simulink model "pd_path_sg"  (R2013b)
settings: Solver=ode45  StartTime=0.0  StopTime=10  RelTol=1e-3
undefined symbols (not defined in the file or in its folder): A, A2, B, C, D, EVAL, i, output_samp_bcoef, PCIN, reg_pk_lim, reg_plim, reg_scale, reg_sr_lim, reg_staclr, reg_txgain, THIS_DATE, W, X, Z
undefined symbols (not defined in the file): lut_address, lut_address_s5, reg_dltap
libraries: xbsIndex_r4 x3819, lut_ram_vhdl x32
(part 10 of 31)

== system pd_path_sg/gmp_model_B/cmp_mul5 ==
  x : Inport
  coef : Inport  Port=2
  pcin_i : Inport  Port=3
  pcin_q : Inport  Port=4
  Convert{10,12,15..16} (4 alike) : xbsIndex_r4/Convert  gui_display_data_type=Fixed-point  arith_type="Signed  (2's comp)"  n_bits=30  bin_pt=0  float_type=Single  exp_bits=8  fraction_bits=24  quantization=Truncate  overflow=Wrap  en=off  latency=0  pipeline=off  dbl_ovrd=off  block_type=convert
  Convert{11,13..14,17} (4 alike) : xbsIndex_r4/Convert  gui_display_data_type=Fixed-point  arith_type="Signed  (2's comp)"  n_bits=18  bin_pt=0  float_type=Single  exp_bits=8  fraction_bits=24  quantization=Truncate  overflow=Wrap  en=off  latency=0  pipeline=off  dbl_ovrd=off  block_type=convert
  "DSP48E2 " : xbsIndex_r4/DSP48E2   use_a=Direct from A Port  use_b=Direct from B Port  addsub_mode=ONE48  xl_useadderonly=off  xl_dynamicmult=off  preaddinsel=A  amultsel=A  bmultsel=B  enable_d=off  reset_preg=off  auto_reset_pr=RESET  pattern_from_creg=1  pattern='000000000000'  mask_from_creg=1  pattern_mask='000000000000'  rnd='000000000000'  widexor=off  xormode=1  use_op=on  use_creg=off  rst_all=off  en_all=off  use_pcin=on  use_carrycascin=off  use_multsignin=off  use_carryout=off  use_patterndetect=off  use_patternbdetect=off  use_overflow=off  use_underflow=off  use_acout=off  use_bcout=off  use_pcout=on  use_multsignout=off  use_carrycascout=off  pipeline_a=2  pipeline_b=2  pipeline_acout=1  pipeline_bcout=1  pipeline_c=on  pipeline_p=on  pipeline_mult=on  pipeline_opmode=on  pipeline_alumode=on  pipeline_carryin=on  pipeline_carryinsel=on  dreg=off  adreg=off  register_inmode=on  rst_a=off  rst_b=off  rst_c=off  rst_mult=off  rst_p=off  rst_carry_in=off  rst_alumode=off  rst_ctrl=off  reset_port_d=off  reset_port_inmode=off  en_a1=off  en_a2=off  en_b1=off  en_b2=off  en_c=off  en_mult=off  en_p=off  en_carry_in=off  en_alumode=off  en_multcarryin=off  en_ctrl=off  enable_port_regd=off  enable_port_regad=off  enable_port_reginmode=off  alumode_inverted=off  alumode_inverted_value='0000'  is_carryin_inverted=off  inmode_inverted=off  inmode_inverted_value='00000'  opmode_inverted=off  opmode_inverted_value='000000000'  is_rstallcarryin_inverted=off  is_rstalumode_inverted=off  is_rsta_inverted=off  is_rstb_inverted=off  is_rstc_inverted=off  is_rstd_inverted=off  is_rstctrl_inverted=off  is_rstinmode_inverted=off  is_rstm_inverted=off  is_rstp_inverted=off  use_synth_model=off  is_clk_inverted=false  block_type=dsp48e2
  DSP48E2 1 : xbsIndex_r4/DSP48E2   use_a=Direct from A Port  use_b=Direct from B Port  addsub_mode=ONE48  xl_useadderonly=off  xl_dynamicmult=off  preaddinsel=A  amultsel=A  bmultsel=B  enable_d=off  reset_preg=off  auto_reset_pr=RESET  pattern_from_creg=1  pattern='000000000000'  mask_from_creg=1  pattern_mask='000000000000'  rnd='000000000000'  widexor=off  xormode=1  use_op=on  use_creg=off  rst_all=off  en_all=off  use_pcin=on  use_carrycascin=off  use_multsignin=off  use_carryout=off  use_patterndetect=off  use_patternbdetect=off  use_overflow=off  use_underflow=off  use_acout=off  use_bcout=off  use_pcout=on  use_multsignout=off  use_carrycascout=off  pipeline_a=1  pipeline_b=1  pipeline_acout=1  pipeline_bcout=1  pipeline_c=on  pipeline_p=on  pipeline_mult=on  pipeline_opmode=on  pipeline_alumode=on  pipeline_carryin=on  pipeline_carryinsel=on  dreg=off  adreg=off  register_inmode=on  rst_a=off  rst_b=off  rst_c=off  rst_mult=off  rst_p=off  rst_carry_in=off  rst_alumode=off  rst_ctrl=off  reset_port_d=off  reset_port_inmode=off  en_a1=off  en_a2=off  en_b1=off  en_b2=off  en_c=off  en_mult=off  en_p=off  en_carry_in=off  en_alumode=off  en_multcarryin=off  en_ctrl=off  enable_port_regd=off  enable_port_regad=off  enable_port_reginmode=off  alumode_inverted=off  alumode_inverted_value='0000'  is_carryin_inverted=off  inmode_inverted=off  inmode_inverted_value='00000'  opmode_inverted=off  opmode_inverted_value='000000000'  is_rstallcarryin_inverted=off  is_rstalumode_inverted=off  is_rsta_inverted=off  is_rstb_inverted=off  is_rstc_inverted=off  is_rstd_inverted=off  is_rstctrl_inverted=off  is_rstinmode_inverted=off  is_rstm_inverted=off  is_rstp_inverted=off  use_synth_model=off  is_clk_inverted=false  block_type=dsp48e2
  DSP48E2 2 : xbsIndex_r4/DSP48E2   use_a=Direct from A Port  use_b=Direct from B Port  addsub_mode=ONE48  xl_useadderonly=off  xl_dynamicmult=off  preaddinsel=A  amultsel=A  bmultsel=B  enable_d=off  reset_preg=off  auto_reset_pr=RESET  pattern_from_creg=1  pattern='000000000000'  mask_from_creg=1  pattern_mask='000000000000'  rnd='000000000000'  widexor=off  xormode=1  use_op=on  use_creg=off  rst_all=off  en_all=off  use_pcin=on  use_carrycascin=off  use_multsignin=off  use_carryout=off  use_patterndetect=off  use_patternbdetect=off  use_overflow=off  use_underflow=off  use_acout=off  use_bcout=off  use_pcout=on  use_multsignout=off  use_carrycascout=off  pipeline_a=2  pipeline_b=2  pipeline_acout=1  pipeline_bcout=1  pipeline_c=on  pipeline_p=on  pipeline_mult=on  pipeline_opmode=on  pipeline_alumode=on  pipeline_carryin=on  pipeline_carryinsel=on  dreg=off  adreg=off  register_inmode=on  rst_a=off  rst_b=off  rst_c=off  rst_mult=off  rst_p=off  rst_carry_in=off  rst_alumode=off  rst_ctrl=off  reset_port_d=off  reset_port_inmode=off  en_a1=off  en_a2=off  en_b1=off  en_b2=off  en_c=off  en_mult=off  en_p=off  en_carry_in=off  en_alumode=off  en_multcarryin=off  en_ctrl=off  enable_port_regd=off  enable_port_regad=off  enable_port_reginmode=off  alumode_inverted=off  alumode_inverted_value='0000'  is_carryin_inverted=off  inmode_inverted=off  inmode_inverted_value='00000'  opmode_inverted=off  opmode_inverted_value='000000000'  is_rstallcarryin_inverted=off  is_rstalumode_inverted=off  is_rsta_inverted=off  is_rstb_inverted=off  is_rstc_inverted=off  is_rstd_inverted=off  is_rstctrl_inverted=off  is_rstinmode_inverted=off  is_rstm_inverted=off  is_rstp_inverted=off  use_synth_model=off  is_clk_inverted=false  block_type=dsp48e2
  DSP48E2 3 : xbsIndex_r4/DSP48E2   use_a=Direct from A Port  use_b=Direct from B Port  addsub_mode=ONE48  xl_useadderonly=off  xl_dynamicmult=off  preaddinsel=A  amultsel=A  bmultsel=B  enable_d=off  reset_preg=off  auto_reset_pr=RESET  pattern_from_creg=1  pattern='000000000000'  mask_from_creg=1  pattern_mask='000000000000'  rnd='000000000000'  widexor=off  xormode=1  use_op=on  use_creg=off  rst_all=off  en_all=off  use_pcin=on  use_carrycascin=off  use_multsignin=off  use_carryout=off  use_patterndetect=off  use_patternbdetect=off  use_overflow=off  use_underflow=off  use_acout=off  use_bcout=off  use_pcout=on  use_multsignout=off  use_carrycascout=off  pipeline_a=1  pipeline_b=1  pipeline_acout=1  pipeline_bcout=1  pipeline_c=on  pipeline_p=on  pipeline_mult=on  pipeline_opmode=on  pipeline_alumode=on  pipeline_carryin=on  pipeline_carryinsel=on  dreg=off  adreg=off  register_inmode=on  rst_a=off  rst_b=off  rst_c=off  rst_mult=off  rst_p=off  rst_carry_in=off  rst_alumode=off  rst_ctrl=off  reset_port_d=off  reset_port_inmode=off  en_a1=off  en_a2=off  en_b1=off  en_b2=off  en_c=off  en_mult=off  en_p=off  en_carry_in=off  en_alumode=off  en_multcarryin=off  en_ctrl=off  enable_port_regd=off  enable_port_regad=off  enable_port_reginmode=off  alumode_inverted=off  alumode_inverted_value='0000'  is_carryin_inverted=off  inmode_inverted=off  inmode_inverted_value='00000'  opmode_inverted=off  opmode_inverted_value='000000000'  is_rstallcarryin_inverted=off  is_rstalumode_inverted=off  is_rsta_inverted=off  is_rstb_inverted=off  is_rstc_inverted=off  is_rstd_inverted=off  is_rstctrl_inverted=off  is_rstinmode_inverted=off  is_rstm_inverted=off  is_rstp_inverted=off  use_synth_model=off  is_clk_inverted=false  block_type=dsp48e2
  Delay{1..4} (4 alike) : xbsIndex_r4/Delay  rst=off  infoeditControl=Selection of Reset will increase slice count due to use of real FFs and instead of SRLs  en=off  latency=10  reg_retiming=off  dbl_ovrd=off  block_type=delay
      settings: infoedit=Hardware notes: A delay line is a chain, each link of which is an SRL16 or SRL32 followed by a flip-flop.
  Demux : Demux  Outputs=2
  Demux1 : Demux  Outputs=2
  Null_p : xbsIndex_r4/Constant  const=0  gui_display_data_type=Fixed-point  arith_type=Unsigned  n_bits=16  bin_pt=0  preci_type=Single  exp_width=8  frac_width=24  explicit_period=off  period=1  equ=P=C  opselect=C  inp2=PCIN>>17  opr=+  inp1=P  carry=CIN  dbl_ovrd=off  block_type=constant
  Null_p1 : xbsIndex_r4/Constant  const=0  gui_display_data_type=Fixed-point  arith_type=Unsigned  n_bits=16  bin_pt=0  preci_type=Single  exp_width=8  frac_width=24  explicit_period=off  period=1  equ=P=C  opselect=C  inp2=PCIN>>17  opr=+  inp1=P  carry=CIN  dbl_ovrd=off  block_type=constant
  Opmode : xbsIndex_r4/Opmode  device=DSP48E2  equ=P=PCIN+(A*B)  operation=PCIN + A*B  inmode_0_3=D+A2  inmode_1_3=A*B  preaddinsel=A  amultsel=A  bmultsel=B  inmode_0=A2  inmode_4=B2  logicinstr=X + W + Z  z_mux=0  xy_mux=A*B  w_mux=RND  carry=0  dbl_ovrd=off  operand=+  x_mux=P  block_type=opmode
  Opmode1 : xbsIndex_r4/Opmode  device=DSP48E2  equ=P=PCIN-(A*B)  operation=Custom  inmode_0_3=D+A2  inmode_1_3=A*B  preaddinsel=A  amultsel=A  bmultsel=B  inmode_0=A2  inmode_4=B2  logicinstr=Z - (X + W)  z_mux=PCIN  xy_mux=A*B  w_mux=0  carry=0  dbl_ovrd=off  operand=+  x_mux=P  block_type=opmode
  Opmode2 : xbsIndex_r4/Opmode  device=DSP48E2  equ=P=PCIN+(A*B)  operation=Custom  inmode_0_3=D+A2  inmode_1_3=A*B  preaddinsel=A  amultsel=A  bmultsel=B  inmode_0=A2  inmode_4=B2  logicinstr=X + W + Z  z_mux=PCIN  xy_mux=A*B  w_mux=0  carry=0  dbl_ovrd=off  operand=+  x_mux=P  block_type=opmode
  Opmode3 : xbsIndex_r4/Opmode  device=DSP48E2  equ=P=PCIN+(A*B)  operation=PCIN + A*B  inmode_0_3=D+A2  inmode_1_3=A*B  preaddinsel=A  amultsel=A  bmultsel=B  inmode_0=A2  inmode_4=B2  logicinstr=X + W + Z  z_mux=PCIN  xy_mux=A*B  w_mux=0  carry=0  dbl_ovrd=off  operand=+  x_mux=P  block_type=opmode
  Terminator{,1..3} (4 alike) : Terminator
  no_route : Outport
  no_route1 : Outport  Port=2
  pcout_i : Outport  Port=3
  pcout_q : Outport  Port=4
  wires:
  Null_p1/1 -> no_route1/1
  Null_p/1 -> no_route/1
  Opmode1/1 -> "DSP48E2 "/4
  Opmode2/1 -> DSP48E2 2/4
  Opmode3/1 -> DSP48E2 3/4
  Opmode/1 -> DSP48E2 1/4
  Delay4/1 -> Convert17/1, Convert13/1
  Delay3/1 -> Convert11/1, Convert14/1
  Delay1/1 -> Convert15/1, Convert12/1
  Delay2/1 -> Convert16/1, Convert10/1
  coef/1 -> Demux1/1
  x/1 -> Demux/1
  Convert12/1 -> "DSP48E2 "/1
  Convert13/1 -> "DSP48E2 "/2
  Convert10/1 -> DSP48E2 1/1
  Convert14/1 -> DSP48E2 1/2
  DSP48E2 1/2 -> "DSP48E2 "/3
  Convert16/1 -> DSP48E2 2/1
  Convert17/1 -> DSP48E2 2/2
  Convert15/1 -> DSP48E2 3/1
  Convert11/1 -> DSP48E2 3/2
  DSP48E2 3/2 -> DSP48E2 2/3
  Demux1/1 -> Delay2/1
  Demux1/2 -> Delay1/1
  Demux/1 -> Delay3/1
  Demux/2 -> Delay4/1
  DSP48E2 1/1 -> Terminator/1
  DSP48E2 3/1 -> Terminator1/1
  DSP48E2 2/2 -> pcout_q/1
  "DSP48E2 "/2 -> pcout_i/1
  "DSP48E2 "/1 -> Terminator2/1
  DSP48E2 2/1 -> Terminator3/1
  pcin_i/1 -> DSP48E2 1/3
  pcin_q/1 -> DSP48E2 3/3

== system pd_path_sg/gmp_model_B/cmp_mul6 ==
  x : Inport
  coef : Inport  Port=2
  pcin_i : Inport  Port=3
  pcin_q : Inport  Port=4
  Convert{10,12,15..16} (4 alike) : xbsIndex_r4/Convert  gui_display_data_type=Fixed-point  arith_type="Signed  (2's comp)"  n_bits=30  bin_pt=0  float_type=Single  exp_bits=8  fraction_bits=24  quantization=Truncate  overflow=Wrap  en=off  latency=0  pipeline=off  dbl_ovrd=off  block_type=convert
  Convert{11,13..14,17} (4 alike) : xbsIndex_r4/Convert  gui_display_data_type=Fixed-point  arith_type="Signed  (2's comp)"  n_bits=18  bin_pt=0  float_type=Single  exp_bits=8  fraction_bits=24  quantization=Truncate  overflow=Wrap  en=off  latency=0  pipeline=off  dbl_ovrd=off  block_type=convert
  "DSP48E2 " : xbsIndex_r4/DSP48E2   use_a=Direct from A Port  use_b=Direct from B Port  addsub_mode=ONE48  xl_useadderonly=off  xl_dynamicmult=off  preaddinsel=A  amultsel=A  bmultsel=B  enable_d=off  reset_preg=off  auto_reset_pr=RESET  pattern_from_creg=1  pattern='000000000000'  mask_from_creg=1  pattern_mask='000000000000'  rnd='000000000000'  widexor=off  xormode=1  use_op=on  use_creg=off  rst_all=off  en_all=off  use_pcin=on  use_carrycascin=off  use_multsignin=off  use_carryout=off  use_patterndetect=off  use_patternbdetect=off  use_overflow=off  use_underflow=off  use_acout=off  use_bcout=off  use_pcout=on  use_multsignout=off  use_carrycascout=off  pipeline_a=2  pipeline_b=2  pipeline_acout=1  pipeline_bcout=1  pipeline_c=on  pipeline_p=on  pipeline_mult=on  pipeline_opmode=on  pipeline_alumode=on  pipeline_carryin=on  pipeline_carryinsel=on  dreg=off  adreg=off  register_inmode=on  rst_a=off  rst_b=off  rst_c=off  rst_mult=off  rst_p=off  rst_carry_in=off  rst_alumode=off  rst_ctrl=off  reset_port_d=off  reset_port_inmode=off  en_a1=off  en_a2=off  en_b1=off  en_b2=off  en_c=off  en_mult=off  en_p=off  en_carry_in=off  en_alumode=off  en_multcarryin=off  en_ctrl=off  enable_port_regd=off  enable_port_regad=off  enable_port_reginmode=off  alumode_inverted=off  alumode_inverted_value='0000'  is_carryin_inverted=off  inmode_inverted=off  inmode_inverted_value='00000'  opmode_inverted=off  opmode_inverted_value='000000000'  is_rstallcarryin_inverted=off  is_rstalumode_inverted=off  is_rsta_inverted=off  is_rstb_inverted=off  is_rstc_inverted=off  is_rstd_inverted=off  is_rstctrl_inverted=off  is_rstinmode_inverted=off  is_rstm_inverted=off  is_rstp_inverted=off  use_synth_model=off  is_clk_inverted=false  block_type=dsp48e2
  DSP48E2 1 : xbsIndex_r4/DSP48E2   use_a=Direct from A Port  use_b=Direct from B Port  addsub_mode=ONE48  xl_useadderonly=off  xl_dynamicmult=off  preaddinsel=A  amultsel=A  bmultsel=B  enable_d=off  reset_preg=off  auto_reset_pr=RESET  pattern_from_creg=1  pattern='000000000000'  mask_from_creg=1  pattern_mask='000000000000'  rnd='000000000000'  widexor=off  xormode=1  use_op=on  use_creg=off  rst_all=off  en_all=off  use_pcin=on  use_carrycascin=off  use_multsignin=off  use_carryout=off  use_patterndetect=off  use_patternbdetect=off  use_overflow=off  use_underflow=off  use_acout=off  use_bcout=off  use_pcout=on  use_multsignout=off  use_carrycascout=off  pipeline_a=1  pipeline_b=1  pipeline_acout=1  pipeline_bcout=1  pipeline_c=on  pipeline_p=on  pipeline_mult=on  pipeline_opmode=on  pipeline_alumode=on  pipeline_carryin=on  pipeline_carryinsel=on  dreg=off  adreg=off  register_inmode=on  rst_a=off  rst_b=off  rst_c=off  rst_mult=off  rst_p=off  rst_carry_in=off  rst_alumode=off  rst_ctrl=off  reset_port_d=off  reset_port_inmode=off  en_a1=off  en_a2=off  en_b1=off  en_b2=off  en_c=off  en_mult=off  en_p=off  en_carry_in=off  en_alumode=off  en_multcarryin=off  en_ctrl=off  enable_port_regd=off  enable_port_regad=off  enable_port_reginmode=off  alumode_inverted=off  alumode_inverted_value='0000'  is_carryin_inverted=off  inmode_inverted=off  inmode_inverted_value='00000'  opmode_inverted=off  opmode_inverted_value='000000000'  is_rstallcarryin_inverted=off  is_rstalumode_inverted=off  is_rsta_inverted=off  is_rstb_inverted=off  is_rstc_inverted=off  is_rstd_inverted=off  is_rstctrl_inverted=off  is_rstinmode_inverted=off  is_rstm_inverted=off  is_rstp_inverted=off  use_synth_model=off  is_clk_inverted=false  block_type=dsp48e2
  DSP48E2 2 : xbsIndex_r4/DSP48E2   use_a=Direct from A Port  use_b=Direct from B Port  addsub_mode=ONE48  xl_useadderonly=off  xl_dynamicmult=off  preaddinsel=A  amultsel=A  bmultsel=B  enable_d=off  reset_preg=off  auto_reset_pr=RESET  pattern_from_creg=1  pattern='000000000000'  mask_from_creg=1  pattern_mask='000000000000'  rnd='000000000000'  widexor=off  xormode=1  use_op=on  use_creg=off  rst_all=off  en_all=off  use_pcin=on  use_carrycascin=off  use_multsignin=off  use_carryout=off  use_patterndetect=off  use_patternbdetect=off  use_overflow=off  use_underflow=off  use_acout=off  use_bcout=off  use_pcout=on  use_multsignout=off  use_carrycascout=off  pipeline_a=2  pipeline_b=2  pipeline_acout=1  pipeline_bcout=1  pipeline_c=on  pipeline_p=on  pipeline_mult=on  pipeline_opmode=on  pipeline_alumode=on  pipeline_carryin=on  pipeline_carryinsel=on  dreg=off  adreg=off  register_inmode=on  rst_a=off  rst_b=off  rst_c=off  rst_mult=off  rst_p=off  rst_carry_in=off  rst_alumode=off  rst_ctrl=off  reset_port_d=off  reset_port_inmode=off  en_a1=off  en_a2=off  en_b1=off  en_b2=off  en_c=off  en_mult=off  en_p=off  en_carry_in=off  en_alumode=off  en_multcarryin=off  en_ctrl=off  enable_port_regd=off  enable_port_regad=off  enable_port_reginmode=off  alumode_inverted=off  alumode_inverted_value='0000'  is_carryin_inverted=off  inmode_inverted=off  inmode_inverted_value='00000'  opmode_inverted=off  opmode_inverted_value='000000000'  is_rstallcarryin_inverted=off  is_rstalumode_inverted=off  is_rsta_inverted=off  is_rstb_inverted=off  is_rstc_inverted=off  is_rstd_inverted=off  is_rstctrl_inverted=off  is_rstinmode_inverted=off  is_rstm_inverted=off  is_rstp_inverted=off  use_synth_model=off  is_clk_inverted=false  block_type=dsp48e2
  DSP48E2 3 : xbsIndex_r4/DSP48E2   use_a=Direct from A Port  use_b=Direct from B Port  addsub_mode=ONE48  xl_useadderonly=off  xl_dynamicmult=off  preaddinsel=A  amultsel=A  bmultsel=B  enable_d=off  reset_preg=off  auto_reset_pr=RESET  pattern_from_creg=1  pattern='000000000000'  mask_from_creg=1  pattern_mask='000000000000'  rnd='000000000000'  widexor=off  xormode=1  use_op=on  use_creg=off  rst_all=off  en_all=off  use_pcin=on  use_carrycascin=off  use_multsignin=off  use_carryout=off  use_patterndetect=off  use_patternbdetect=off  use_overflow=off  use_underflow=off  use_acout=off  use_bcout=off  use_pcout=on  use_multsignout=off  use_carrycascout=off  pipeline_a=1  pipeline_b=1  pipeline_acout=1  pipeline_bcout=1  pipeline_c=on  pipeline_p=on  pipeline_mult=on  pipeline_opmode=on  pipeline_alumode=on  pipeline_carryin=on  pipeline_carryinsel=on  dreg=off  adreg=off  register_inmode=on  rst_a=off  rst_b=off  rst_c=off  rst_mult=off  rst_p=off  rst_carry_in=off  rst_alumode=off  rst_ctrl=off  reset_port_d=off  reset_port_inmode=off  en_a1=off  en_a2=off  en_b1=off  en_b2=off  en_c=off  en_mult=off  en_p=off  en_carry_in=off  en_alumode=off  en_multcarryin=off  en_ctrl=off  enable_port_regd=off  enable_port_regad=off  enable_port_reginmode=off  alumode_inverted=off  alumode_inverted_value='0000'  is_carryin_inverted=off  inmode_inverted=off  inmode_inverted_value='00000'  opmode_inverted=off  opmode_inverted_value='000000000'  is_rstallcarryin_inverted=off  is_rstalumode_inverted=off  is_rsta_inverted=off  is_rstb_inverted=off  is_rstc_inverted=off  is_rstd_inverted=off  is_rstctrl_inverted=off  is_rstinmode_inverted=off  is_rstm_inverted=off  is_rstp_inverted=off  use_synth_model=off  is_clk_inverted=false  block_type=dsp48e2
  Delay{1..4} (4 alike) : xbsIndex_r4/Delay  rst=off  infoeditControl=Selection of Reset will increase slice count due to use of real FFs and instead of SRLs  en=off  latency=12  reg_retiming=off  dbl_ovrd=off  block_type=delay
      settings: infoedit=Hardware notes: A delay line is a chain, each link of which is an SRL16 or SRL32 followed by a flip-flop.
  Demux : Demux  Outputs=2
  Demux1 : Demux  Outputs=2
  Null_p : xbsIndex_r4/Constant  const=0  gui_display_data_type=Fixed-point  arith_type=Unsigned  n_bits=16  bin_pt=0  preci_type=Single  exp_width=8  frac_width=24  explicit_period=off  period=1  equ=P=C  opselect=C  inp2=PCIN>>17  opr=+  inp1=P  carry=CIN  dbl_ovrd=off  block_type=constant
  Null_p1 : xbsIndex_r4/Constant  const=0  gui_display_data_type=Fixed-point  arith_type=Unsigned  n_bits=16  bin_pt=0  preci_type=Single  exp_width=8  frac_width=24  explicit_period=off  period=1  equ=P=C  opselect=C  inp2=PCIN>>17  opr=+  inp1=P  carry=CIN  dbl_ovrd=off  block_type=constant
  Opmode : xbsIndex_r4/Opmode  device=DSP48E2  equ=P=PCIN+(A*B)  operation=PCIN + A*B  inmode_0_3=D+A2  inmode_1_3=A*B  preaddinsel=A  amultsel=A  bmultsel=B  inmode_0=A2  inmode_4=B2  logicinstr=X + W + Z  z_mux=0  xy_mux=A*B  w_mux=RND  carry=0  dbl_ovrd=off  operand=+  x_mux=P  block_type=opmode
  Opmode1 : xbsIndex_r4/Opmode  device=DSP48E2  equ=P=PCIN-(A*B)  operation=Custom  inmode_0_3=D+A2  inmode_1_3=A*B  preaddinsel=A  amultsel=A  bmultsel=B  inmode_0=A2  inmode_4=B2  logicinstr=Z - (X + W)  z_mux=PCIN  xy_mux=A*B  w_mux=0  carry=0  dbl_ovrd=off  operand=+  x_mux=P  block_type=opmode
  Opmode2 : xbsIndex_r4/Opmode  device=DSP48E2  equ=P=PCIN+(A*B)  operation=Custom  inmode_0_3=D+A2  inmode_1_3=A*B  preaddinsel=A  amultsel=A  bmultsel=B  inmode_0=A2  inmode_4=B2  logicinstr=X + W + Z  z_mux=PCIN  xy_mux=A*B  w_mux=0  carry=0  dbl_ovrd=off  operand=+  x_mux=P  block_type=opmode
  Opmode3 : xbsIndex_r4/Opmode  device=DSP48E2  equ=P=PCIN+(A*B)  operation=PCIN + A*B  inmode_0_3=D+A2  inmode_1_3=A*B  preaddinsel=A  amultsel=A  bmultsel=B  inmode_0=A2  inmode_4=B2  logicinstr=X + W + Z  z_mux=PCIN  xy_mux=A*B  w_mux=0  carry=0  dbl_ovrd=off  operand=+  x_mux=P  block_type=opmode
  Terminator : Terminator
  Terminator1 : Terminator
  no_route : Outport
  no_route1 : Outport  Port=2
  iout : Outport  Port=3
  qout : Outport  Port=4
  wires:
  DSP48E2 2/1 -> qout/1
  "DSP48E2 "/1 -> iout/1
  pcin_q/1 -> DSP48E2 3/3
  pcin_i/1 -> DSP48E2 1/3
  DSP48E2 3/1 -> Terminator1/1
  DSP48E2 1/1 -> Terminator/1
  Demux/2 -> Delay4/1
  Demux/1 -> Delay3/1
  Demux1/2 -> Delay1/1
  Demux1/1 -> Delay2/1
  DSP48E2 3/2 -> DSP48E2 2/3
  Convert11/1 -> DSP48E2 3/2
  Convert15/1 -> DSP48E2 3/1
  Convert17/1 -> DSP48E2 2/2
  Convert16/1 -> DSP48E2 2/1
  DSP48E2 1/2 -> "DSP48E2 "/3
  Convert14/1 -> DSP48E2 1/2
  Convert10/1 -> DSP48E2 1/1
  Convert13/1 -> "DSP48E2 "/2
  Convert12/1 -> "DSP48E2 "/1
  x/1 -> Demux/1
  coef/1 -> Demux1/1
  Delay2/1 -> Convert10/1, Convert16/1
  Delay1/1 -> Convert12/1, Convert15/1
  Delay3/1 -> Convert14/1, Convert11/1
  Delay4/1 -> Convert13/1, Convert17/1
  Opmode/1 -> DSP48E2 1/4
  Opmode3/1 -> DSP48E2 3/4
  Opmode2/1 -> DSP48E2 2/4
  Opmode1/1 -> "DSP48E2 "/4
  Null_p/1 -> no_route/1
  Null_p1/1 -> no_route1/1

== system pd_path_sg/input_samp_a/input_samp ==
  In1 : Inport
  Delay{1..5} (5 alike) : xbsIndex_r4/Delay  rst=off  infoeditControl=Selection of Reset will increase slice count due to use of real FFs and instead of SRLs  en=off  latency=4  reg_retiming=off  dbl_ovrd=off  block_type=delay
      settings: infoedit=Hardware notes: A delay line is a chain, each link of which is an SRL16 or SRL32 followed by a flip-flop.
  mult : Subsystem
  ori_seq : Outport
  interp_seq : Outport  Port=2
  wires:
  In1/1 -> mult/1(in1), Delay1/1
  Delay1/1 -> Delay2/1, mult/3(in3)
  Delay2/1 -> Delay3/1, mult/5(in5)
  mult/1(Out1) -> interp_seq/1
  Delay5/1 -> mult/2(in2)
  Delay3/1 -> mult/6(in6), Delay4/1
  Delay4/1 -> ori_seq/1, mult/4(in4), Delay5/1

== system pd_path_sg/input_samp_b/input_samp ==
  In1 : Inport
  Delay{1..5} (5 alike) : xbsIndex_r4/Delay  rst=off  infoeditControl=Selection of Reset will increase slice count due to use of real FFs and instead of SRLs  en=off  latency=4  reg_retiming=off  dbl_ovrd=off  block_type=delay
      settings: infoedit=Hardware notes: A delay line is a chain, each link of which is an SRL16 or SRL32 followed by a flip-flop.
  mult : Subsystem
  ori_seq : Outport
  interp_seq : Outport  Port=2
  wires:
  Delay4/1 -> Delay5/1, mult/4(in4), ori_seq/1
  Delay3/1 -> Delay4/1, mult/6(in6)
  Delay5/1 -> mult/2(in2)
  mult/1(Out1) -> interp_seq/1
  Delay2/1 -> mult/5(in5), Delay3/1
  Delay1/1 -> mult/3(in3), Delay2/1
  In1/1 -> Delay1/1, mult/1(in1)

== system pd_path_sg/other_regs/perbus_reg ==
  addr : Inport
  din : Inport  Port=2
  we : Inport  Port=3
  Logical1 : xbsIndex_r4/Logical  logical_function=AND  inputs=2  en=off  latency=0  precision=Full  arith_type=Unsigned  n_bits=16  bin_pt=0  align_bp=on  dbl_ovrd=off  block_type=logical
  REG_ADDR : xbsIndex_r4/Constant  const=hex2dec('140')  gui_display_data_type=Fixed-point  arith_type=Unsigned  n_bits=12  bin_pt=0  preci_type=Single  exp_width=8  frac_width=24  explicit_period=off  period=1  equ=P=C  opselect=C  inp2=PCIN>>17  opr=+  inp1=P  carry=CIN  dbl_ovrd=off  block_type=constant
  Register1 : xbsIndex_r4/Register  init=0  rst=off  en=on  dbl_ovrd=off  block_type=register
  Register2 : xbsIndex_r4/Register  init=0  rst=off  en=on  dbl_ovrd=off  block_type=register
  Relational2 : xbsIndex_r4/Relational  mode=a=b  op_type=Bool  en=off  latency=0  dbl_ovrd=off  block_type=relational
  b[3-1] : xbsIndex_r4/Slice  nbits=4  boolean_output=off  mode=Lower Bit Location + Width  bit1=0  base1=MSB of Input  bit0=0  base0=LSB of Input  dbl_ovrd=off  block_type=slice
  b[4] : xbsIndex_r4/Slice  nbits=1  boolean_output=off  mode=Lower Bit Location + Width  bit1=0  base1=MSB of Input  bit0=4  base0=LSB of Input  dbl_ovrd=off  block_type=slice
  band : Outport
  lut_active : Outport  Port=2
  wires:
  we/1 -> Logical1/1
  addr/1 -> Relational2/1
  Relational2/1 -> Logical1/2
  REG_ADDR/1 -> Relational2/2
  din/1 -> b[3-1]/1, b[4]/1
  b[3-1]/1 -> Register1/1
  b[4]/1 -> Register2/1
  Logical1/1 -> Register1/2, Register2/2
  Register1/1 -> lut_active/1
  Register2/1 -> band/1

== system pd_path_sg/output_sw_A/add_switch ==
  chi : Inport
  x : Inport  Port=2
  d : Inport  Port=3
  on0 : Inport  Port=4
  on1 : Inport  Port=5
  AddSub1 : xbsIndex_r4/AddSub  mode=Addition  use_carryin=off  use_carryout=off  en=off  latency=1  precision=User Defined  arith_type="Signed  (2's comp)"  n_bits=17  bin_pt=0  quantization=Truncate  overflow=Wrap  use_behavioral_HDL=off  hw_selection=Fabric  pipelined=off  dbl_ovrd=off  block_type=addsub
  AddSub2 : xbsIndex_r4/AddSub  mode=Addition  use_carryin=off  use_carryout=off  en=off  latency=1  precision=User Defined  arith_type="Signed  (2's comp)"  n_bits=17  bin_pt=0  quantization=Truncate  overflow=Wrap  use_behavioral_HDL=off  hw_selection=Fabric  pipelined=off  dbl_ovrd=off  block_type=addsub
  Constant : xbsIndex_r4/Constant  const=0  gui_display_data_type=Fixed-point  arith_type=Signed (2's comp)  n_bits=17  bin_pt=0  preci_type=Single  exp_width=8  frac_width=24  explicit_period=off  period=1  equ=P=C  opselect=C  inp2=PCIN>>17  opr=+  inp1=P  carry=CIN  dbl_ovrd=off  block_type=constant
  Constant1 : xbsIndex_r4/Constant  const=0  gui_display_data_type=Fixed-point  arith_type=Signed (2's comp)  n_bits=17  bin_pt=0  preci_type=Single  exp_width=8  frac_width=24  explicit_period=off  period=1  equ=P=C  opselect=C  inp2=PCIN>>17  opr=+  inp1=P  carry=CIN  dbl_ovrd=off  block_type=constant
  Delay : xbsIndex_r4/Delay  rst=off  infoeditControl=Selection of Reset will increase slice count due to use of real FFs and instead of SRLs  en=off  latency=delaytaps+1  reg_retiming=off  dbl_ovrd=off  block_type=delay
      settings: infoedit=Hardware notes: A delay line is a chain, each link of which is an SRL16 or SRL32 followed by a flip-flop.
  Delay1 : xbsIndex_r4/Delay  rst=off  infoeditControl=Selection of Reset will increase slice count due to use of real FFs and instead of SRLs  en=off  latency=delaytaps+1  reg_retiming=off  dbl_ovrd=off  block_type=delay
      settings: infoedit=Hardware notes: A delay line is a chain, each link of which is an SRL16 or SRL32 followed by a flip-flop.
  Delay2 : xbsIndex_r4/Delay  rst=off  infoeditControl=Selection of Reset will increase slice count due to use of real FFs and instead of SRLs  en=off  latency=delaytaps  reg_retiming=off  dbl_ovrd=off  block_type=delay
      settings: infoedit=Hardware notes: A delay line is a chain, each link of which is an SRL16 or SRL32 followed by a flip-flop.
  Delay3 : xbsIndex_r4/Delay  rst=off  infoeditControl=Selection of Reset will increase slice count due to use of real FFs and instead of SRLs  en=off  latency=delaytaps  reg_retiming=off  dbl_ovrd=off  block_type=delay
      settings: infoedit=Hardware notes: A delay line is a chain, each link of which is an SRL16 or SRL32 followed by a flip-flop.
  Delay4 : xbsIndex_r4/Delay  rst=off  infoeditControl=Selection of Reset will increase slice count due to use of real FFs and instead of SRLs  en=off  latency=delaytaps  reg_retiming=off  dbl_ovrd=off  block_type=delay
      settings: infoedit=Hardware notes: A delay line is a chain, each link of which is an SRL16 or SRL32 followed by a flip-flop.
  Delay5 : xbsIndex_r4/Delay  rst=off  infoeditControl=Selection of Reset will increase slice count due to use of real FFs and instead of SRLs  en=off  latency=2  reg_retiming=off  dbl_ovrd=off  block_type=delay
      settings: infoedit=Hardware notes: A delay line is a chain, each link of which is an SRL16 or SRL32 followed by a flip-flop.
  Demux1 : Demux  Outputs=2
  Demux2 : Demux  Outputs=2
  Mux : xbsIndex_r4/Mux  inputs=2  en=off  latency=1  precision=Full  arith_type=Unsigned  n_bits=16  bin_pt=14  quantization=Truncate  overflow=Wrap  dbl_ovrd=off  block_type=mux
  Mux1 : xbsIndex_r4/Mux  inputs=2  en=off  latency=0  precision=Full  arith_type=Unsigned  n_bits=16  bin_pt=14  quantization=Truncate  overflow=Wrap  dbl_ovrd=off  block_type=mux
  Mux2 : xbsIndex_r4/Mux  inputs=2  en=off  latency=1  precision=Full  arith_type=Unsigned  n_bits=16  bin_pt=14  quantization=Truncate  overflow=Wrap  dbl_ovrd=off  block_type=mux
  Mux3 : Mux  Inputs=2
  cho : Outport
  y : Outport  Port=2
  wires:
  Constant/1 -> Mux/2
  on0/1 -> Mux1/2
  on1/1 -> Mux1/3
  chi/1 -> Delay4/1
  x/1 -> Demux1/1
  d/1 -> Demux2/1
  Demux1/1 -> Delay/1
  Demux1/2 -> Delay1/1
  Constant1/1 -> Mux2/2
  Demux2/1 -> Delay2/1
  Demux2/2 -> Delay3/1
  Mux/1 -> AddSub1/2
  Mux2/1 -> AddSub2/2
  AddSub1/1 -> Mux3/1
  AddSub2/1 -> Mux3/2
  Mux3/1 -> y/1
  Delay/1 -> AddSub1/1
  Delay1/1 -> AddSub2/1
  Delay2/1 -> Mux/3
  Delay3/1 -> Mux2/3
  Delay4/1 -> Delay5/1, Mux1/1
  Delay5/1 -> cho/1
  Mux1/1 -> Mux2/1, Mux/1

== system pd_path_sg/output_sw_A/ch_split ==
  per : Inport
  chnsel : Inport  Port=2
  Bus Creator : BusCreator  Inputs=3
  Bus Creator1 : BusCreator  Inputs=3
  Bus Selector : BusSelector  OutputSignals=addr,din,we
  Constant : xbsIndex_r4/Constant  const=0  gui_display_data_type=Boolean  arith_type=Boolean  n_bits=16  bin_pt=14  preci_type=Single  exp_width=8  frac_width=24  explicit_period=off  period=1  equ=P=C  opselect=C  inp2=PCIN>>17  opr=+  inp1=P  carry=CIN  dbl_ovrd=off  block_type=constant
  Constant1 : xbsIndex_r4/Constant  const=0  gui_display_data_type=Boolean  arith_type=Boolean  n_bits=16  bin_pt=14  preci_type=Single  exp_width=8  frac_width=24  explicit_period=off  period=1  equ=P=C  opselect=C  inp2=PCIN>>17  opr=+  inp1=P  carry=CIN  dbl_ovrd=off  block_type=constant
  Mux : xbsIndex_r4/Mux  inputs=2  en=off  latency=0  precision=Full  arith_type=Unsigned  n_bits=16  bin_pt=14  quantization=Truncate  overflow=Wrap  dbl_ovrd=off  block_type=mux
  Mux1 : xbsIndex_r4/Mux  inputs=2  en=off  latency=0  precision=Full  arith_type=Unsigned  n_bits=16  bin_pt=14  quantization=Truncate  overflow=Wrap  dbl_ovrd=off  block_type=mux
  per0 : Outport
  per1 : Outport  Port=2
  wires:
  per/1 -> Bus Selector/1
  Bus Selector/1 -> Bus Creator1/1, Bus Creator/1  "<addr>"
  Bus Selector/2 -> Bus Creator1/2, Bus Creator/2  "<din>"
  chnsel/1 -> Mux1/1, Mux/1
  Constant/1 -> Mux/3
  Bus Selector/3 -> Mux1/3, Mux/2  "<we>"
  Constant1/1 -> Mux1/2
  Mux1/1 -> Bus Creator1/3  "we"
  Bus Creator1/1 -> per1/1
  Mux/1 -> Bus Creator/3  "we"
  Bus Creator/1 -> per0/1

== system pd_path_sg/output_sw_A/config_regs0 ==
  per : Inport
  rst : Inport  Port=2
  B0 : xbsIndex_r4/Slice  nbits=1  boolean_output=on  mode=Lower Bit Location + Width  bit1=0  base1=MSB of Input  bit0=0  base0=LSB of Input  dbl_ovrd=off  block_type=slice
  B1 : xbsIndex_r4/Slice  nbits=1  boolean_output=on  mode=Lower Bit Location + Width  bit1=0  base1=MSB of Input  bit0=1  base0=LSB of Input  dbl_ovrd=off  block_type=slice
  B2 : xbsIndex_r4/Slice  nbits=16  boolean_output=off  mode=Lower Bit Location + Width  bit1=0  base1=MSB of Input  bit0=0  base0=LSB of Input  dbl_ovrd=off  block_type=slice
  Bus Selector : BusSelector  OutputSignals=addr,din,we
  Slice : xbsIndex_r4/Slice  nbits=16  boolean_output=off  mode=Lower Bit Location + Width  bit1=0  base1=MSB of Input  bit0=0  base0=LSB of Input  dbl_ovrd=off  block_type=slice
  Slice1 : xbsIndex_r4/Slice  nbits=16  boolean_output=off  mode=Lower Bit Location + Width  bit1=0  base1=MSB of Input  bit0=0  base0=LSB of Input  dbl_ovrd=off  block_type=slice
  perbus_reg : Subsystem
  perbus_reg1 : Subsystem
  perbus_reg2 : Subsystem
  perbus_reg3 : Subsystem
  sr_lim : Outport
  pk_lim : Outport  Port=2
  alarm_clr : Outport  Port=3
  pd_on : Outport  Port=4
  tx_gain : Outport  Port=5
  wires:
  Slice1/1 -> pk_lim/1
  Slice/1 -> sr_lim/1
  perbus_reg1/1(q) -> Slice1/1
  perbus_reg/1(q) -> Slice/1
  Bus Selector/3 -> perbus_reg3/3(we), perbus_reg2/3(we), perbus_reg1/3(we), perbus_reg/3(we)  "<we>"
  Bus Selector/2 -> perbus_reg1/2(din), perbus_reg3/2(din), perbus_reg2/2(din), perbus_reg/2(din)  "<din>"
  Bus Selector/1 -> perbus_reg3/1(addr), perbus_reg2/1(addr), perbus_reg1/1(addr), perbus_reg/1(addr)  "<addr>"
  per/1 -> Bus Selector/1
  perbus_reg2/1(q) -> B1/1, B0/1
  B0/1 -> alarm_clr/1
  B1/1 -> pd_on/1
  perbus_reg3/1(q) -> B2/1
  B2/1 -> tx_gain/1
  rst/1 -> perbus_reg2/4(rst), perbus_reg3/4(rst)

== system pd_path_sg/output_sw_A/config_regs1 ==
  per : Inport
  rst : Inport  Port=2
  B0 : xbsIndex_r4/Slice  nbits=1  boolean_output=on  mode=Lower Bit Location + Width  bit1=0  base1=MSB of Input  bit0=0  base0=LSB of Input  dbl_ovrd=off  block_type=slice
  B1 : xbsIndex_r4/Slice  nbits=1  boolean_output=on  mode=Lower Bit Location + Width  bit1=0  base1=MSB of Input  bit0=1  base0=LSB of Input  dbl_ovrd=off  block_type=slice
  B2 : xbsIndex_r4/Slice  nbits=16  boolean_output=off  mode=Lower Bit Location + Width  bit1=0  base1=MSB of Input  bit0=0  base0=LSB of Input  dbl_ovrd=off  block_type=slice
  Bus Selector : BusSelector  OutputSignals=addr,din,we
  Slice : xbsIndex_r4/Slice  nbits=16  boolean_output=off  mode=Lower Bit Location + Width  bit1=0  base1=MSB of Input  bit0=0  base0=LSB of Input  dbl_ovrd=off  block_type=slice
  Slice1 : xbsIndex_r4/Slice  nbits=16  boolean_output=off  mode=Lower Bit Location + Width  bit1=0  base1=MSB of Input  bit0=0  base0=LSB of Input  dbl_ovrd=off  block_type=slice
  perbus_reg : Subsystem
  perbus_reg1 : Subsystem
  perbus_reg2 : Subsystem
  perbus_reg3 : Subsystem
  sr_lim : Outport
  pk_lim : Outport  Port=2
  alarm_clr : Outport  Port=3
  pd_on : Outport  Port=4
  tx_gain : Outport  Port=5
  wires:
  rst/1 -> perbus_reg3/4(rst), perbus_reg2/4(rst)
  B2/1 -> tx_gain/1
  perbus_reg3/1(q) -> B2/1
  B1/1 -> pd_on/1
  B0/1 -> alarm_clr/1
  perbus_reg2/1(q) -> B0/1, B1/1
  per/1 -> Bus Selector/1
  Bus Selector/1 -> perbus_reg/1(addr), perbus_reg1/1(addr), perbus_reg2/1(addr), perbus_reg3/1(addr)  "<addr>"
  Bus Selector/2 -> perbus_reg/2(din), perbus_reg2/2(din), perbus_reg3/2(din), perbus_reg1/2(din)  "<din>"
  Bus Selector/3 -> perbus_reg/3(we), perbus_reg1/3(we), perbus_reg2/3(we), perbus_reg3/3(we)  "<we>"
  perbus_reg/1(q) -> Slice/1
  perbus_reg1/1(q) -> Slice1/1
  Slice/1 -> sr_lim/1
  Slice1/1 -> pk_lim/1

== system pd_path_sg/output_sw_A/detect_i ==
  chi : Inport
  x : Inport  Port=2
  d : Inport  Port=3
  pk0 : Inport  Port=4
  pk1 : Inport  Port=5
  sr0 : Inport  Port=6
  sr1 : Inport  Port=7
  Absolute : xbsIndex_r4/Absolute  precision=User Defined  arith_type="Signed  (2's comp)"  n_bits=9  bin_pt=0  quantization=Truncate  overflow=Wrap  en=off  latency=0  dbl_ovrd=off  block_type=abs
  Absolute1 : xbsIndex_r4/Absolute  precision=User Defined  arith_type="Signed  (2's comp)"  n_bits=9  bin_pt=0  quantization=Truncate  overflow=Wrap  en=off  latency=0  dbl_ovrd=off  block_type=abs
  AddSub1 : xbsIndex_r4/AddSub  mode=Addition  use_carryin=off  use_carryout=off  en=off  latency=1  precision=User Defined  arith_type="Signed  (2's comp)"  n_bits=9  bin_pt=0  quantization=Truncate  overflow=Wrap  use_behavioral_HDL=off  hw_selection=Fabric  pipelined=off  dbl_ovrd=off  block_type=addsub
  AddSub2 : xbsIndex_r4/AddSub  mode=Subtraction  use_carryin=off  use_carryout=off  en=off  latency=1  precision=User Defined  arith_type="Signed  (2's comp)"  n_bits=9  bin_pt=0  quantization=Truncate  overflow=Wrap  use_behavioral_HDL=off  hw_selection=Fabric  pipelined=off  dbl_ovrd=off  block_type=addsub
  Delay : xbsIndex_r4/Delay  rst=off  infoeditControl=Selection of Reset will increase slice count due to use of real FFs and instead of SRLs  en=off  latency=2  reg_retiming=off  dbl_ovrd=off  block_type=delay
      settings: infoedit=Hardware notes: A delay line is a chain, each link of which is an SRL16 or SRL32 followed by a flip-flop.
  Delay1 : xbsIndex_r4/Delay  rst=off  infoeditControl=Selection of Reset will increase slice count due to use of real FFs and instead of SRLs  en=off  latency=2  reg_retiming=off  dbl_ovrd=off  block_type=delay
      settings: infoedit=Hardware notes: A delay line is a chain, each link of which is an SRL16 or SRL32 followed by a flip-flop.
  Mux : xbsIndex_r4/Mux  inputs=2  en=off  latency=1  precision=Full  arith_type=Unsigned  n_bits=16  bin_pt=14  quantization=Truncate  overflow=Wrap  dbl_ovrd=off  block_type=mux
  Mux1 : xbsIndex_r4/Mux  inputs=2  en=off  latency=1  precision=Full  arith_type=Unsigned  n_bits=16  bin_pt=14  quantization=Truncate  overflow=Wrap  dbl_ovrd=off  block_type=mux
  Relational : xbsIndex_r4/Relational  mode=a>b  op_type=Bool  en=off  latency=1  dbl_ovrd=off  block_type=relational
  Relational1 : xbsIndex_r4/Relational  mode=a>b  op_type=Bool  en=off  latency=1  dbl_ovrd=off  block_type=relational
  cut8bit : Subsystem
  cut8bit1 : Subsystem
  cut8bit2 : Subsystem
  cut8bit3 : Subsystem
  cut8bit4 : Subsystem
  cut8bit5 : Subsystem
  cho : Outport
  pk_alarm : Outport  Port=2
  sr_alarm : Outport  Port=3
  wires:
  x/1 -> cut8bit/1(d)
  d/1 -> cut8bit1/1(d)
  pk0/1 -> cut8bit2/1(d)
  AddSub1/1 -> Absolute/1
  Absolute/1 -> Relational/1
  Relational/1 -> pk_alarm/1
  cut8bit2/1(q) -> Mux/2
  pk1/1 -> cut8bit3/1(d)
  Mux/1 -> Relational/2
  cut8bit1/1(q) -> AddSub2/1, Delay/1, AddSub1/2
  chi/1 -> Mux/1, Delay1/1, Mux1/1
  cut8bit4/1(q) -> Mux1/2
  cut8bit5/1(q) -> Mux1/3
  Delay/1 -> AddSub2/2
  Absolute1/1 -> Relational1/1
  AddSub2/1 -> Absolute1/1
  Mux1/1 -> Relational1/2
  sr0/1 -> cut8bit4/1(d)
  sr1/1 -> cut8bit5/1(d)
  Relational1/1 -> sr_alarm/1
  Delay1/1 -> cho/1
  cut8bit/1(q) -> AddSub1/1
  cut8bit3/1(q) -> Mux/3

== system pd_path_sg/output_sw_A/detect_q ==
  chi : Inport
  x : Inport  Port=2
  d : Inport  Port=3
  pk0 : Inport  Port=4
  pk1 : Inport  Port=5
  sr0 : Inport  Port=6
  sr1 : Inport  Port=7
  Absolute : xbsIndex_r4/Absolute  precision=User Defined  arith_type="Signed  (2's comp)"  n_bits=9  bin_pt=0  quantization=Truncate  overflow=Wrap  en=off  latency=0  dbl_ovrd=off  block_type=abs
  Absolute1 : xbsIndex_r4/Absolute  precision=User Defined  arith_type="Signed  (2's comp)"  n_bits=9  bin_pt=0  quantization=Truncate  overflow=Wrap  en=off  latency=0  dbl_ovrd=off  block_type=abs
  AddSub1 : xbsIndex_r4/AddSub  mode=Addition  use_carryin=off  use_carryout=off  en=off  latency=1  precision=User Defined  arith_type="Signed  (2's comp)"  n_bits=9  bin_pt=0  quantization=Truncate  overflow=Wrap  use_behavioral_HDL=off  hw_selection=Fabric  pipelined=off  dbl_ovrd=off  block_type=addsub
  AddSub2 : xbsIndex_r4/AddSub  mode=Subtraction  use_carryin=off  use_carryout=off  en=off  latency=1  precision=User Defined  arith_type="Signed  (2's comp)"  n_bits=9  bin_pt=0  quantization=Truncate  overflow=Wrap  use_behavioral_HDL=off  hw_selection=Fabric  pipelined=off  dbl_ovrd=off  block_type=addsub
  Delay : xbsIndex_r4/Delay  rst=off  infoeditControl=Selection of Reset will increase slice count due to use of real FFs and instead of SRLs  en=off  latency=2  reg_retiming=off  dbl_ovrd=off  block_type=delay
      settings: infoedit=Hardware notes: A delay line is a chain, each link of which is an SRL16 or SRL32 followed by a flip-flop.
  Delay1 : xbsIndex_r4/Delay  rst=off  infoeditControl=Selection of Reset will increase slice count due to use of real FFs and instead of SRLs  en=off  latency=2  reg_retiming=off  dbl_ovrd=off  block_type=delay
      settings: infoedit=Hardware notes: A delay line is a chain, each link of which is an SRL16 or SRL32 followed by a flip-flop.
  Mux : xbsIndex_r4/Mux  inputs=2  en=off  latency=1  precision=Full  arith_type=Unsigned  n_bits=16  bin_pt=14  quantization=Truncate  overflow=Wrap  dbl_ovrd=off  block_type=mux
  Mux1 : xbsIndex_r4/Mux  inputs=2  en=off  latency=1  precision=Full  arith_type=Unsigned  n_bits=16  bin_pt=14  quantization=Truncate  overflow=Wrap  dbl_ovrd=off  block_type=mux
  Relational : xbsIndex_r4/Relational  mode=a>b  op_type=Bool  en=off  latency=1  dbl_ovrd=off  block_type=relational
  Relational1 : xbsIndex_r4/Relational  mode=a>b  op_type=Bool  en=off  latency=1  dbl_ovrd=off  block_type=relational
  cut8bit : Subsystem
  cut8bit1 : Subsystem
  cut8bit2 : Subsystem
  cut8bit3 : Subsystem
  cut8bit4 : Subsystem
  cut8bit5 : Subsystem
  cho : Outport
  pk_alarm : Outport  Port=2
  sr_alarm : Outport  Port=3
  wires:
  cut8bit3/1(q) -> Mux/3
  cut8bit/1(q) -> AddSub1/1
  Delay1/1 -> cho/1
  Relational1/1 -> sr_alarm/1
  sr1/1 -> cut8bit5/1(d)
  sr0/1 -> cut8bit4/1(d)
  Mux1/1 -> Relational1/2
  AddSub2/1 -> Absolute1/1
  Absolute1/1 -> Relational1/1
  Delay/1 -> AddSub2/2
  cut8bit5/1(q) -> Mux1/3
  cut8bit4/1(q) -> Mux1/2
  chi/1 -> Mux1/1, Delay1/1, Mux/1
  cut8bit1/1(q) -> AddSub1/2, Delay/1, AddSub2/1
  Mux/1 -> Relational/2
  pk1/1 -> cut8bit3/1(d)
  cut8bit2/1(q) -> Mux/2
  Relational/1 -> pk_alarm/1
  Absolute/1 -> Relational/1
  AddSub1/1 -> Absolute/1
  pk0/1 -> cut8bit2/1(d)
  d/1 -> cut8bit1/1(d)
  x/1 -> cut8bit/1(d)

== system pd_path_sg/output_sw_A/on_status ==
  chi : Inport
  pki_alarm : Inport  Port=2
  sri_alarm : Inport  Port=3
  pkq_alarm : Inport  Port=4
  srq_alarm : Inport  Port=5
  clr0 : Inport  Port=6
  clr1 : Inport  Port=7
  on0 : Inport  Port=8
  on1 : Inport  Port=9
  chnsel : Inport  Port=10
  Constant : xbsIndex_r4/Constant  const=0  gui_display_data_type=Boolean  arith_type=Boolean  n_bits=1  bin_pt=0  preci_type=Single  exp_width=8  frac_width=24  explicit_period=off  period=1  equ=P=C  opselect=C  inp2=PCIN>>17  opr=+  inp1=P  carry=CIN  dbl_ovrd=off  block_type=constant
  Constant{1..2,4..5} (4 alike) : xbsIndex_r4/Constant  const=1  gui_display_data_type=Boolean  arith_type=Boolean  n_bits=1  bin_pt=0  preci_type=Single  exp_width=8  frac_width=24  explicit_period=off  period=1  equ=P=C  opselect=C  inp2=PCIN>>17  opr=+  inp1=P  carry=CIN  dbl_ovrd=off  block_type=constant
  Constant3 : xbsIndex_r4/Constant  const=0  gui_display_data_type=Boolean  arith_type=Boolean  n_bits=1  bin_pt=0  preci_type=Single  exp_width=8  frac_width=24  explicit_period=off  period=1  equ=P=C  opselect=C  inp2=PCIN>>17  opr=+  inp1=P  carry=CIN  dbl_ovrd=off  block_type=constant
  Inverter : xbsIndex_r4/Inverter  en=off  latency=0  dbl_ovrd=off  block_type=inv
  Inverter1 : xbsIndex_r4/Inverter  en=off  latency=0  dbl_ovrd=off  block_type=inv
  Logical{,1..2,4,6..7} (6 alike) : xbsIndex_r4/Logical  logical_function=OR  inputs=2  en=off  latency=0  precision=Full  arith_type=Unsigned  n_bits=16  bin_pt=0  align_bp=on  dbl_ovrd=off  block_type=logical
  Logical3 : xbsIndex_r4/Logical  logical_function=AND  inputs=2  en=off  latency=0  precision=Full  arith_type=Unsigned  n_bits=16  bin_pt=0  align_bp=on  dbl_ovrd=off  block_type=logical
  Logical5 : xbsIndex_r4/Logical  logical_function=AND  inputs=2  en=off  latency=0  precision=Full  arith_type=Unsigned  n_bits=16  bin_pt=0  align_bp=on  dbl_ovrd=off  block_type=logical
  Mux{,1..3} (4 alike) : xbsIndex_r4/Mux  inputs=2  en=off  latency=0  precision=Full  arith_type=Unsigned  n_bits=16  bin_pt=14  quantization=Truncate  overflow=Wrap  dbl_ovrd=off  block_type=mux
  Mux4 : xbsIndex_r4/Mux  inputs=2  en=off  latency=1  precision=Full  arith_type=Unsigned  n_bits=16  bin_pt=14  quantization=Truncate  overflow=Wrap  dbl_ovrd=off  block_type=mux
  Mux5 : xbsIndex_r4/Mux  inputs=2  en=off  latency=1  precision=Full  arith_type=Unsigned  n_bits=16  bin_pt=14  quantization=Truncate  overflow=Wrap  dbl_ovrd=off  block_type=mux
  pk0 : xbsIndex_r4/Register  init=0  rst=on  en=on  dbl_ovrd=off  block_type=register
  pk1 : xbsIndex_r4/Register  init=0  rst=on  en=on  dbl_ovrd=off  block_type=register
  sr0 : xbsIndex_r4/Register  init=0  rst=on  en=on  dbl_ovrd=off  block_type=register
  sr1 : xbsIndex_r4/Register  init=0  rst=on  en=on  dbl_ovrd=off  block_type=register
  pk_status : Outport
  sr_status : Outport  Port=2
  sw0 : Outport  Port=3
  sw1 : Outport  Port=4
  wires:
  pki_alarm/1 -> Logical6/1, Logical/1
  pkq_alarm/1 -> Logical6/2, Logical/2
  Constant/1 -> Mux1/2, Mux/3
  Mux/1 -> pk0/3
  Constant1/1 -> pk0/1
  Constant2/1 -> pk1/1
  Mux1/1 -> pk1/3
  Logical1/1 -> Mux2/2
  Constant3/1 -> Mux2/3, Mux3/2
  Mux2/1 -> sr0/3
  Constant4/1 -> sr0/1
  Constant5/1 -> sr1/1
  Mux3/1 -> sr1/3
  sri_alarm/1 -> Logical7/1, Logical1/1
  srq_alarm/1 -> Logical7/2, Logical1/2
  pk0/1 -> Mux4/2, Logical2/1
  sr0/1 -> Mux5/2, Logical2/2
  Logical2/1 -> Inverter/1
  Inverter/1 -> Logical3/2
  Logical4/1 -> Inverter1/1
  Inverter1/1 -> Logical5/2
  pk1/1 -> Mux4/3, Logical4/1
  sr1/1 -> Mux5/3, Logical4/2
  Logical3/1 -> sw0/1
  Logical5/1 -> sw1/1
  chi/1 -> Mux2/1, Mux3/1, Mux1/1, Mux/1
  chnsel/1 -> Mux5/1, Mux4/1
  Mux4/1 -> pk_status/1
  Mux5/1 -> sr_status/1
  clr0/1 -> sr0/2, pk0/2
  clr1/1 -> sr1/2, pk1/2
  Logical6/1 -> Mux1/3
  Logical7/1 -> Mux3/3
  on1/1 -> Logical5/1
  on0/1 -> Logical3/1
  Logical/1 -> Mux/2
